simulink model "adder_tree_test"  (Simulink 7.0)
settings: Solver=VariableStepDiscrete  SolverMode=SingleTasking  StartTime=0.0  StopTime=256  RelTol=1e-3
libraries: xbsIndex_r4 x22
settings Model: Creator=User  LastModifiedBy=User
settings DebuggingCC: SaveWithDisabledLinksMsg=none

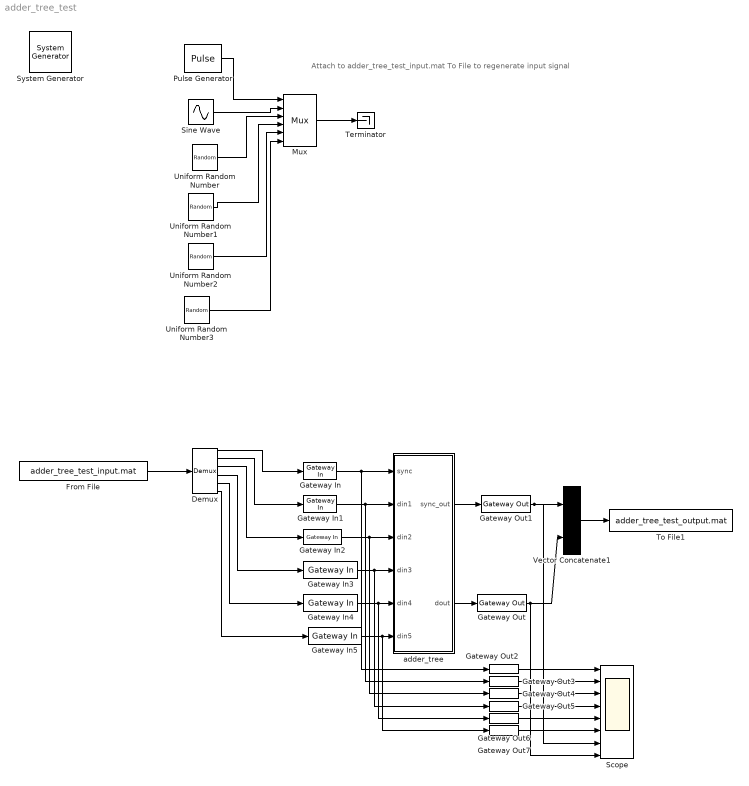
== system adder_tree_test ==
  note: Attach to adder_tree_test_input.mat To File
      | to regenerate input signal
  " System Generator" : xbsIndex_r4/ System Generator  Tag=genX  SystemSampleTime=-1  xilinxfamily=Virtex4  part=xc4vsx35  speed=-10  package=ff668  synthesis_tool=XST  clock_wrapper=Clock Enables  directory=./netlist  testbench=off  simulink_period=1  sysclk_period=10  dcm_input_clock_period=100  incr_netlist=off  trim_vbits=Everywhere in SubSystem  dbl_ovrd=According to Block Masks  core_generation=According to Block Masks  run_coregen=off  deprecated_control=off  eval_field=0  block_type=sysgen
      settings: block_version=8.2.02
  Demux : Demux  Outputs=6
  From File : FromFile  FileName=adder_tree_test_input.mat  SampleTime=1
  Gateway In : xbsIndex_r4/Gateway In  arith_type=Boolean  n_bits=25  bin_pt=0  quantization="Round  (unbiased: +/- Inf)"  overflow=Saturate  period=1  dbl_ovrd=off  timing_constraint=None  locs_specified=off  LOCs={}  block_type=gatewayin
      settings: infoedit="Gateway in block.  Converts inputs of type Simulink integer, double and fixed point to  Xilinx fixed point type.<P><P>Hardware notes:  In hardware these blocks become top level input ports."  block_version=10.1.1
  Gateway In1 : xbsIndex_r4/Gateway In  arith_type="Signed  (2's comp)"  n_bits=8  bin_pt=0  quantization=Truncate  overflow=Saturate  period=1  dbl_ovrd=off  timing_constraint=None  locs_specified=off  LOCs={}  block_type=gatewayin
      settings: infoedit="Gateway in block.  Converts inputs of type Simulink integer, double and fixed point to  Xilinx fixed point type.<P><P>Hardware notes:  In hardware these blocks become top level input ports."  block_version=10.1.1
  Gateway In{2..5} (4 alike) : xbsIndex_r4/Gateway In  arith_type="Signed  (2's comp)"  n_bits=8  bin_pt=0  quantization="Round  (unbiased: +/- Inf)"  overflow=Saturate  period=1  dbl_ovrd=off  timing_constraint=None  locs_specified=off  LOCs={}  block_type=gatewayin
      settings: infoedit="Gateway in block.  Converts inputs of type Simulink integer, double and fixed point to  Xilinx fixed point type.<P><P>Hardware notes:  In hardware these blocks become top level input ports."  block_version=10.1.1
  Gateway Out{,1..7} (8 alike) : xbsIndex_r4/Gateway Out  hdl_port=on  timing_constraint=None  locs_specified=off  LOCs={}  block_type=gatewayout
      settings: infoedit="Gateway out block.  Converts Xilinx fixed point inputs into ouputs of type Simulink integer, double, or fixed point.<P><P>Hardware notes:  In hardware these blocks become top level output ports or are discarded, depending on how they are configured."  block_version=10.1.1
  Mux : Mux  Inputs=6
  Pulse Generator : DiscretePulseGenerator  Period=32  PhaseDelay=10
  Scope : Scope  NumInputPorts=8
      settings: TimeRange=1200  YMin=0~-200~-200~-200~0~-400~-5~-5  YMax=1~200~200~200~1~400~5~5
  Sine Wave : Sin  SineType=Sample based  Amplitude=128  Samples=256  SampleTime=1
  Terminator : Terminator
  To File1 : ToFile  Filename=adder_tree_test_output.mat  MatrixName=output
  Uniform Random Number : UniformRandomNumber  Minimum=-128  Maximum=127  SampleTime=1
  Uniform Random Number1 : UniformRandomNumber  Minimum=-128  Maximum=127  Seed=1  SampleTime=1
  Uniform Random Number2 : UniformRandomNumber  Minimum=-128  Maximum=127  Seed=2  SampleTime=1
  Uniform Random Number3 : UniformRandomNumber  Minimum=-128  Maximum=127  Seed=3  SampleTime=1
  Vector Concatenate1 : Concatenate  Mode=Vector
  adder_tree : Subsystem  AncestorBlock=casper_library/Misc/adder_tree  mask(adder_tree){n_inputs=5, latency=3}
      mask prompts: n_inputs "Number of Inputs"; latency "Add Latency"
      mask help: Sums all inputs using a tree of adds and delays.
      mask init:
      | adder_tree_init(gcb, ...
      |     'n_inputs', n_inputs, ...
      |     'latency', latency);
      settings: AttributesFormatString=latency 9
      mask Help: eval('xlWeb([getenv(''MLIB_ROOT''), ''\doc\htmlblocks\sp_adder_tree\sp_adder_tree.html''])')
  wires:
  Pulse Generator/1 -> Mux/1
  Gateway In/1 -> Gateway Out2/1, adder_tree/1(sync)
  Gateway In1/1 -> Gateway Out3/1, adder_tree/2(din1)
  Gateway In2/1 -> Gateway Out4/1, adder_tree/3(din2)
  Gateway In3/1 -> Gateway Out5/1, adder_tree/4(din3)
  adder_tree/1(sync_out) -> Gateway Out1/1
  adder_tree/2(dout) -> Gateway Out/1
  Gateway Out1/1 -> Vector Concatenate1/1, Scope/7
  Gateway Out/1 -> Vector Concatenate1/2, Scope/8
  Vector Concatenate1/1 -> To File1/1
  Demux/1 -> Gateway In/1
  Demux/2 -> Gateway In1/1
  Demux/3 -> Gateway In2/1
  Demux/4 -> Gateway In3/1
  Mux/1 -> Terminator/1
  Sine Wave/1 -> Mux/2
  Gateway Out2/1 -> Scope/1
  Gateway Out3/1 -> Scope/2
  Gateway Out4/1 -> Scope/3
  Gateway Out5/1 -> Scope/4
  Uniform Random Number/1 -> Mux/3
  Uniform Random Number1/1 -> Mux/4
  Uniform Random Number2/1 -> Mux/5
  Demux/5 -> Gateway In4/1
  Gateway In4/1 -> adder_tree/5(din4), Gateway Out6/1
  Uniform Random Number3/1 -> Mux/6
  Demux/6 -> Gateway In5/1
  Gateway In5/1 -> adder_tree/6(din5), Gateway Out7/1
  Gateway Out6/1 -> Scope/5
  Gateway Out7/1 -> Scope/6
  From File/1 -> Demux/1

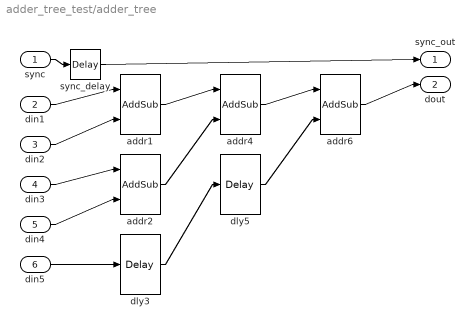
== system adder_tree_test/adder_tree ==
  sync : Inport  OutDataType=sfix(16)  OutScaling=2^0
  din1 : Inport  Port=2  OutDataType=sfix(16)  OutScaling=2^0
  din2 : Inport  Port=3  OutDataType=sfix(16)  OutScaling=2^0
  din3 : Inport  Port=4  OutDataType=sfix(16)  OutScaling=2^0
  din4 : Inport  Port=5
  din5 : Inport  Port=6
  addr1 : xbsIndex_r4/AddSub  mode=Addition  use_carryin=off  use_carryout=off  en=off  latency=3  precision=Full  arith_type=Unsigned  n_bits=8  bin_pt=2  quantization=Truncate  overflow=Wrap  dbl_ovrd=off  use_behavioral_HDL=on  pipelined=on  use_rpm=on  block_type=addsub
      settings: xl_area=[0, 0, 0, 0, 0, 0, 0]  block_version=9.1.01
  addr2 : xbsIndex_r4/AddSub  mode=Addition  use_carryin=off  use_carryout=off  en=off  latency=3  precision=Full  arith_type=Unsigned  n_bits=16  bin_pt=14  quantization=Truncate  overflow=Wrap  dbl_ovrd=off  use_behavioral_HDL=off  pipelined=on  use_rpm=on  block_type=addsub
      settings: block_version=10.1.1
  addr4 : xbsIndex_r4/AddSub  mode=Addition  use_carryin=off  use_carryout=off  en=off  latency=3  precision=Full  arith_type=Unsigned  n_bits=16  bin_pt=14  quantization=Truncate  overflow=Wrap  dbl_ovrd=off  use_behavioral_HDL=off  pipelined=on  use_rpm=on  block_type=addsub
      settings: block_version=10.1.1
  addr6 : xbsIndex_r4/AddSub  mode=Addition  use_carryin=off  use_carryout=off  en=off  latency=3  precision=Full  arith_type=Unsigned  n_bits=16  bin_pt=14  quantization=Truncate  overflow=Wrap  dbl_ovrd=off  use_behavioral_HDL=off  pipelined=on  use_rpm=on  block_type=addsub
      settings: block_version=10.1.1
  dly3 : xbsIndex_r4/Delay  en=off  latency=3  dbl_ovrd=off  reg_retiming=off  block_type=delay
      settings: block_version=10.1.1
  dly5 : xbsIndex_r4/Delay  en=off  latency=3  dbl_ovrd=off  reg_retiming=off  block_type=delay
      settings: block_version=10.1.1
  sync_delay : xbsIndex_r4/Delay  en=off  latency=9  dbl_ovrd=off  reg_retiming=off  block_type=delay
      settings: xl_area=[0, 0, 0, 0, 0, 0, 0]  block_version=9.1.01
  sync_out : Outport  OutDataType=sfix(16)  OutScaling=2^0
  dout : Outport  Port=2  OutDataType=sfix(16)  OutScaling=2^0
  wires:
  addr6/1 -> dout/1
  dly5/1 -> addr6/2
  addr4/1 -> addr6/1
  dly3/1 -> dly5/1
  addr2/1 -> addr4/2
  addr1/1 -> addr4/1
  din5/1 -> dly3/1
  din4/1 -> addr2/2
  din3/1 -> addr2/1
  din2/1 -> addr1/2
  din1/1 -> addr1/1
  sync_delay/1 -> sync_out/1
  sync/1 -> sync_delay/1
